simulink model "DAEMOT_Motor"  (R2025a)
settings: Solver=ode15s  StartTime=0.0  StopTime=10.0  RelTol=1e-3
undefined symbols (not defined in the file or in its folder): rev_comms_sink
settings Model: Creator=jmp8430  LastModifiedBy=jmp8430

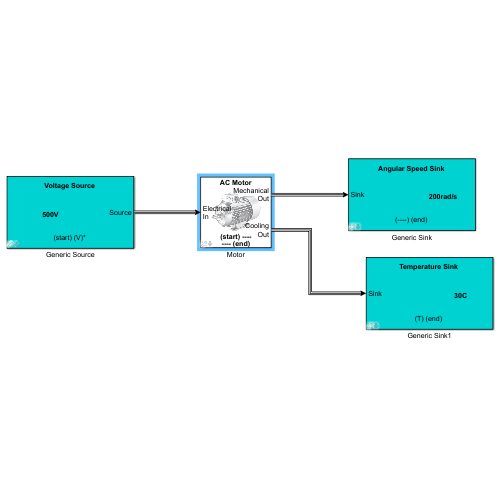
[thumbnail: Simulink's stored preview of the top-level diagram]
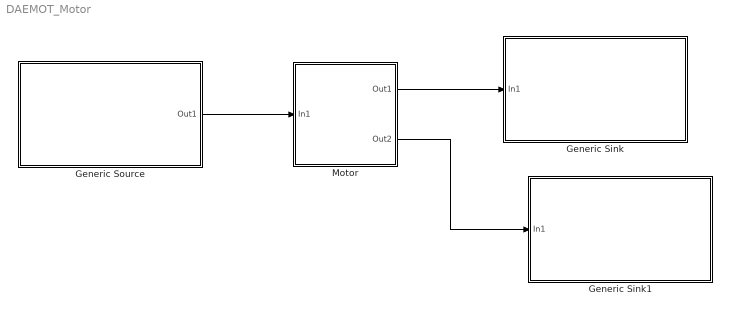
== system DAEMOT_Motor ==
  Generic Sink : Subsystem  AncestorBlock=DAEMOT_Lib/Support Functions/Generic Sink  mask(Effort Sink (Torque)){Stype=Angular Speed Sink, const=on, value=200}
      mask prompts: Stype "Sink Type"; const "Constant Value?"; value "Speed [rad/s]"
      mask help: Used to create a effot sink.
      mask init:
      | h      = get_param(gcb,'handle');   % Get block handle
      | blk    = gcb;
      | hblock = get(h);     % Parse out handles structure
      | 
      | if const == 1;
      |     try delete_block([blk,'/In2'])
      |         delete_unconnected_lines(blk);
      |         add_block('simulink/Sources/Constant',   [blk,'/val'], 'Position', [200,218,230,232]);
      |         add_line(blk,'val/1','Sink1/1','AutoRouting','on');
      |         set_param([blk,'/val'],'Value','value');
      |     end
      |      
      | %     delete_unconnected_lines(blk)
      | else
      |     try delete_block([blk,'/val'])
      |         delete_unconnected_lines(blk);
      |         add_block('simulink/Ports & Subsystems/In1',   [blk,'/In2'], 'Position', [200,218,230,232]);
      |         add_line(blk,'In2/1','Sink1/1','AutoRouting','on');
      |     end
      | end
      | 
      | clear h blk hblock
      settings: CopyFcn=|
      | h      = get_param(gcb,'handle');   % Get block handle
      | blk    = gcb;
      | 
      | set_param(blk, 'LinkStatus', 'inactive')
      | clear h
      | clear blk
      mask TypeOptions Stype: Voltage Sink | Current Sink | Angular Speed Sink | Torque Sink | Temperature Sink | Heat Flow Sink | Pressure Sink | Mass Flow Sink
      mask Callback Stype:
      | mp     = get_param(gcb,'MaskPrompts');
      | h      = get_param(gcb,'handle');   % Get block handle
      | blk    = gcb;
      | hblock = get(h);     % Parse out handles structure
      | 
      | switch get_param(gcb,'Stype')
      |     case 'Voltage Sink'
      |         mp{3} = 'Voltage [V]';
      |     case 'Current Sink'
      |         mp{3} = 'Current [A]';
      |     case 'Angular Speed Sink'
      |         mp{3} = 'Speed [rad/s]';
      |     case 'Torque Sink'
      |         mp{3} = 'Torque [Nm]';
      |     case 'Temperature Sink'
      |         mp{3} = 'Temperature [C]';
      |     case 'Heat Flow Sink'
      |         mp{3} = 'Heat Flow [kW]';
      |     case 'Pressure Sink'
      |         mp{3} = 'Pressure [kPa]';
      |     case 'Mass Flow Sink'
      |         mp{3} = 'Mass Flow [kg/s]';
      | end
      | set_param(gcb,'MaskPrompts',mp);
      | 
      | clear mp h blk hblock
      mask Callback const:
      | en = get_param(gcb,'MaskVisibilities');
      | h      = get_param(gcb,'handle');   % Get block handle
      | blk    = gcb;
      | hblock = get(h);     % Parse out handles structure
      | 
      | switch get_param(gcb,'const')
      |     case 'on'
      |         en{3} = 'on';
      | %         delete_block([blk,'/In1'])
      | 
      |     case 'off'
      |         en{3} = 'off';
      | %         add_block('simulink/Ports & Subsystems/In1',   [blk,'/In1'],'Position',[130    -7   160     7]);         % adding inport
      | 
      | end
      | set_param(gcb,'MaskVisibilities',en);
      | 
      | % hblock.MaskPrompts{3} = 'hello';
      | clear en h blk hblock
      mask Display:
      | text(0.5,0.90,['{\bf',get_param(gcb,'Stype'),'}'],'TexMode','on','horizontalAlignment', 'center')
      | % text(0.5,0.1,['{(T)(end)}'],'TexMode','on','horizontalAlignment', 'center')
      | 
      | type = get_param(gcb,'Stype');
      | switch type
      |         case 'Voltage Sink'
      |             nm = 'Voltage [V]';
      |             id = '(V)';
      |             un = 'V';
      |         case 'Current Sink'
      |             nm = 'Current [A]';
      |             id = '(----)';
      |             un = 'A';
      |         case 'Angular Speed Sink'
      |             nm = 'Speed [rad/s]';
      |             id = '(----)';
      |             un = 'rad/s';
      |         case 'Torque Sink'
      |             nm = 'Torque [Nm]';
      |             id = '(\tau)';
      |             un = 'Nm';
      |         case 'Temperature Sink'
      |             nm = 'Temperature [C]';
      |             id = '(T)';
      |             un = 'C';
      |         case 'Heat Flow Sink'
      |             nm = 'Heat Flow [kW]';
      |             id = '(----)';
      |             un = 'kW';
      |         case 'Pressure Sink'
      |             nm = 'Pressure [kPa]';
      |             id = '(P)';
      |             un = 'kPa';
      |         case 'Mass Flow Sink'
      |             nm = 'Mass Flow [kg/s]';
      |             id = '(----)';
      |             un = 'kg/s';
      | end
      | 
      | if strcmp(get_param(gcb,'const'),'on')
      |     text(0.75,0.500,['{\bf',get_param(gcb,'Value'),un,'}'],'TexMode','on','horizontalAlignment', 'center')
      | else
      |     port_label('input',2,sprintf(['Sink ',nm]));
      | end
      | 
      | 
      | port_label('input',1,'Sink');
      | text(0.5,0.175,['{',id,' (end)}'],'TexMode','on','horizontalAlignment', 'center');
  Generic Sink1 : Subsystem  AncestorBlock=DAEMOT_Lib/Support Functions/Generic Sink  mask(Effort Sink (Torque)){Stype=Temperature Sink, const=on, value=30}
      mask prompts: Stype "Sink Type"; const "Constant Value?"; value "Temperature [C]"
      mask help: Used to create a effot sink.
      mask init: same as DAEMOT_Motor/Generic Sink
      settings: CopyFcn=|
      | h      = get_param(gcb,'handle');   % Get block handle
      | blk    = gcb;
      | 
      | set_param(blk, 'LinkStatus', 'inactive')
      | clear h
      | clear blk
      mask TypeOptions Stype: Voltage Sink | Current Sink | Angular Speed Sink | Torque Sink | Temperature Sink | Heat Flow Sink | Pressure Sink | Mass Flow Sink
      mask Callback Stype:
      | mp     = get_param(gcb,'MaskPrompts');
      | h      = get_param(gcb,'handle');   % Get block handle
      | blk    = gcb;
      | hblock = get(h);     % Parse out handles structure
      | 
      | switch get_param(gcb,'Stype')
      |     case 'Voltage Sink'
      |         mp{3} = 'Voltage [V]';
      |     case 'Current Sink'
      |         mp{3} = 'Current [A]';
      |     case 'Angular Speed Sink'
      |         mp{3} = 'Speed [rad/s]';
      |     case 'Torque Sink'
      |         mp{3} = 'Torque [Nm]';
      |     case 'Temperature Sink'
      |         mp{3} = 'Temperature [C]';
      |     case 'Heat Flow Sink'
      |         mp{3} = 'Heat Flow [kW]';
      |     case 'Pressure Sink'
      |         mp{3} = 'Pressure [kPa]';
      |     case 'Mass Flow Sink'
      |         mp{3} = 'Mass Flow [kg/s]';
      | end
      | set_param(gcb,'MaskPrompts',mp);
      | 
      | clear mp h blk hblock
      mask Callback const:
      | en = get_param(gcb,'MaskVisibilities');
      | h      = get_param(gcb,'handle');   % Get block handle
      | blk    = gcb;
      | hblock = get(h);     % Parse out handles structure
      | 
      | switch get_param(gcb,'const')
      |     case 'on'
      |         en{3} = 'on';
      | %         delete_block([blk,'/In1'])
      | 
      |     case 'off'
      |         en{3} = 'off';
      | %         add_block('simulink/Ports & Subsystems/In1',   [blk,'/In1'],'Position',[130    -7   160     7]);         % adding inport
      | 
      | end
      | set_param(gcb,'MaskVisibilities',en);
      | 
      | % hblock.MaskPrompts{3} = 'hello';
      | clear en h blk hblock
      mask Display:
      | text(0.5,0.90,['{\bf',get_param(gcb,'Stype'),'}'],'TexMode','on','horizontalAlignment', 'center')
      | % text(0.5,0.1,['{(T)(end)}'],'TexMode','on','horizontalAlignment', 'center')
      | 
      | type = get_param(gcb,'Stype');
      | switch type
      |         case 'Voltage Sink'
      |             nm = 'Voltage [V]';
      |             id = '(V)';
      |             un = 'V';
      |         case 'Current Sink'
      |             nm = 'Current [A]';
      |             id = '(----)';
      |             un = 'A';
      |         case 'Angular Speed Sink'
      |             nm = 'Speed [rad/s]';
      |             id = '(----)';
      |             un = 'rad/s';
      |         case 'Torque Sink'
      |             nm = 'Torque [Nm]';
      |             id = '(\tau)';
      |             un = 'Nm';
      |         case 'Temperature Sink'
      |             nm = 'Temperature [C]';
      |             id = '(T)';
      |             un = 'C';
      |         case 'Heat Flow Sink'
      |             nm = 'Heat Flow [kW]';
      |             id = '(----)';
      |             un = 'kW';
      |         case 'Pressure Sink'
      |             nm = 'Pressure [kPa]';
      |             id = '(P)';
      |             un = 'kPa';
      |         case 'Mass Flow Sink'
      |             nm = 'Mass Flow [kg/s]';
      |             id = '(----)';
      |             un = 'kg/s';
      | end
      | 
      | if strcmp(get_param(gcb,'const'),'on')
      |     text(0.75,0.500,['{\bf',get_param(gcb,'Value'),un,'}'],'TexMode','on','horizontalAlignment', 'center')
      | else
      |     port_label('input',2,sprintf(['Sink ',nm]));
      | end
      | 
      | 
      | port_label('input',1,'Sink');
      | text(0.5,0.175,['{',id,' (end)}'],'TexMode','on','horizontalAlignment', 'center');
  Generic Source : Subsystem  AncestorBlock=DAEMOT_Lib/Support Functions/Generic Source  mask(Effort Source (Voltage)){Stype=Voltage Source, const=on, value=500}
      mask prompts: Stype "Source Type"; const "Constant Value?"; value "Voltage [V]"
      mask help: Used to create an effort source.
      mask init:
      | h      = get_param(gcb,'handle');   % Get block handle
      | blk    = gcb;
      | hblock = get(h);     % Parse out handles structure
      | type = get_param(gcb,'Stype');
      |         
      | switch type
      |     case 'Voltage Source'
      |         up = 'current';
      |         dw = 'voltage';
      |     case 'Current Source'
      |         dw = 'current';
      |         up = 'voltage';
      |     case 'Angular Speed Source'
      |         up = 'torque';
      |         dw = 'aspeed';
      |     case 'Torque Source'
      |         dw = 'torque';
      |         up = 'aspeed';
      |     case 'Temperature Source'
      |         up = 'Q_kW';
      |         dw = 'Temp';
      |     case 'Heat Flow Source'
      |         dw = 'Q_kW';
      |         up = 'Temp';
      |     case 'Pressure Source'
      |         up = 'mdot_kgps';
      |         mid= 'T_C';
      |         dw = 'P_kPa';
      |     case 'Mass Flow Source'
      |         up = 'P_kpa';
      |         mid= 'T_C';
      |         dw = 'mdot_kgps';
      |         %up = 'mdot_kgps';
      |         %mid= 'T_C';
      |         %dw = 'P_kPa';
      | end
      | 
      | if (((type(1) == 'P') || (type(1) == 'M')) && (const == 1)) %if constant input (user defined in mask) and need temperature input
      |     
      |     try add_block('simulink/Ports & Subsystems/In1', [blk,'/In2'], 'Position', [200,230,230,245]) %make temperature input
      |         set_param([blk, '/b1'],'Inputs','3');
      |         add_line(blk,'In2/1','b1/3','AutoRouting','on');
      |             
      |         p = get_param([blk,'/In2'],'PortHandles');
      |         l = get_param(p.Outport,'Line');
      |         set_param(l,'Name',mid);
      |     end 
      |     
      |     try delete_block([blk,'/In1'])
      |         delete_unconnected_lines(blk);
      |         
      |         fprintf ("option 1\n");        
      |         
      |         add_block('simulink/Sources/Constant',   [blk,'/val'], 'Position', [200,148,230,162]);
      |         add_line(blk,'val/1','b1/2','AutoRouting','on');
      |         set_param([blk,'/val'],'Value','value');
      |         
      |         p = get_param([blk,'/Constant'],'PortHandles');
      |         l = get_param(p.Outport,'Line');
      |         set_param(l,'Name',up);
      | 
      |         p = get_param([blk,'/val'],'PortHandles');
      |         l = get_param(p.Outport,'Line');
      |         set_param(l,'Name',dw);
      |         
      |     end
      |     p = get_param([blk,'/Constant'],'PortHandles');
      |     l = get_param(p.Outport,'Line');
      | 
      |     if (strcmp(get_param(l,'name'),up)) %If it didn't work and l's name doesn't match what it should, set them again.
      |     else
      |         set_param(l,'Name',up);
      |         
      |         fprintf ("failed strcmp \n");
      |                 
      |         p = get_param([blk,'/val'],'PortHandles');
      |         l = get_param(p.Outport,'Line');
      |         set_param(l,'Name',dw);
      |             
      |         p = get_param([blk,'/In2'],'PortHandles');
      |         l = get_param(p.Outport,'Line');
      |         set_param(l,'Name',mid);
      |     end
      |     
      | elseif ((type(1) == 'P') || (type(1) == 'M')) %if need input port (not user defined in mask) and also need temperature input
      |     
      |     try add_block('simulink/Ports & Subsystems/In1', [blk,'/In2'], 'Position', [200,230,230,245]) %make temperature input
      |         set_param([blk, '/b1'],'Inputs','3');
      |         add_line(blk,'In2/1','b1/3','AutoRouting','on');
      | 
      |         p = get_param([blk,'/In2'],'PortHandles');
      |         l = get_param(p.Outport,'Line');
      |         set_param(l,'Name',mid);
      |     end
      |     
      |     try delete_block([blk,'/val'])
      |         delete_unconnected_lines(blk);
      |         
      |         fprintf ("option 2\n");      
      |         
      |         add_block('simulink/Ports & Subsystems/In1', [blk,'/In1'], 'Position', [200,148,230,162]);
      |         add_line(blk,'In1/1','b1/2','AutoRouting','on');
      |         
      |         p = get_param([blk,'/Constant'],'PortHandles');
      |         l = get_param(p.Outport,'Line');
      |         set_param(l,'Name',up);
      | 
      |         p = get_param([blk,'/In1'],'PortHandles');
      |         l = get_param(p.Outport,'Line');
      |         set_param(l,'Name',dw);
      |         
      |     end
      |     
      |     p = get_param([blk,'/Constant'],'PortHandles');
      |     l = get_param(p.Outport,'Line');
      |     if (strcmp(get_param(l,'name'),up)) %If it didn't work and l's name doesn't match what it should, set them again.
      |     else
      |         set_param(l,'Name',up);
      |         
      |         fprintf ("failed strcmp \n");
      |         
      |         p = get_param([blk,'/In1'],'PortHandles');
      |         l = get_param(p.Outport,'Line');
      |         set_param(l,'Name',dw);
      | 
      |         p = get_param([blk,'/In2'],'PortHandles');
      |         l = get_param(p.Outport,'Line');
      |         set_param(l,'Name',mid);
      |     end
      |     
      | elseif (const == 1) %if constant, user-defined input, but does not need a temperature input port
      |     try delete_block([blk,'/In2']) %delete temperature input
      |         delete_unconnected_lines(blk);
      |         
      |         set_param([blk, '/b1'],'Inputs','2');
      |         fprintf ("delete in2 \n");
      |     end
      |     
      |     try delete_block([blk,'/In1'])
      |         delete_unconnected_lines(blk);
      |         
      |         fprintf ("option 3\n");
      |         
      |         add_block('simulink/Sources/Constant',   [blk,'/val'], 'Position', [200,198,230,212]);
      |         add_line(blk,'val/1','b1/2','AutoRouting','on');
      |         set_param([blk,'/val'],'Value','value');
      |         
      |         p = get_param([blk,'/Constant'],'PortHandles');
      |         l = get_param(p.Outport,'Line');
      |         set_param(l,'Name',up);
      |         
      |         p = get_param([blk,'/val'],'PortHandles');
      |         l = get_param(p.Outport,'Line');
      |         set_param(l,'Name',dw);
      |     end
      |     
      |     p = get_param([blk,'/Constant'],'PortHandles');
      |     l = get_param(p.Outport,'Line');
      |     if (strcmp(get_param(l,'name'),up))
      |     else
      |         set_param(l,'Name',up);
      |         
      |         fprintf ("failed strcmp \n");
      |                 
      |         p = get_param([blk,'/val'],'PortHandles');
      |         l = get_param(p.Outport,'Line');
      |         set_param(l,'Name',dw);
      |     end
      |     
      | else %if need an input port for the input, but not for temperature
      |     try delete_block([blk,'/In2']) %delete temperature input
      |         delete_unconnected_lines(blk);
      |         
      |         set_param([blk, '/b1'],'Inputs','2');
      |         fprintf ("deleted in2 \n");
      |     end    
      |         
      |     try delete_block([blk,'/val'])
      |         delete_unconnected_lines(blk);
      |         
      |         fprintf ("option 4\n");
      |         
      |         add_block('simulink/Ports & Subsystems/In1',   [blk,'/In1'], 'Position', [200,198,230,212]);
      |         add_line(blk,'In1/1','b1/2','AutoRouting','on');
      |         
      |         p = get_param([blk,'/Constant'],'PortHandles');
      |         l = get_param(p.Outport,'Line');
      |         set_param(l,'Name',up);
      | 
      |         p = get_param([blk,'/In1'],'PortHandles');
      |         l = get_param(p.Outport,'Line');
      |         set_param(l,'Name',dw);
      |     end
      |     
      |     p = get_param([blk,'/Constant'],'PortHandles');
      |     l = get_param(p.Outport,'Line');
      |     if (strcmp(get_param(l,'name'),up))
      |     else
      |         set_param(l,'Name',up);
      |         fprintf ("failed strcmp \n");
      |         p = get_param([blk,'/In1'],'PortHandles');
      |         l = get_param(p.Outport,'Line');
      |         set_param(l,'Name',dw);
      |     end
      |     
      | end
      | 
      | 
      | %if const == 1;
      | %    try delete_block([blk,'/In1'])
      | %        delete_unconnected_lines(blk);
      | %        add_block('simulink/Sources/Constant',   [blk,'/val'], 'Position', [200,198,230,212]);
      | %        add_line(blk,'val/1','b1/2','AutoRouting','on');
      | %        set_param([blk,'/val'],'Value','value');
      | 
      | %        p = get_param([blk,'/Constant'],'PortHandles');
      | %        l = get_param(p.Outport,'Line');
      | %        set_param(l,'Name',up);
      |         
      | %        p = get_param([blk,'/val'],'PortHandles');
      | %        l = get_param(p.Outport,'Line');
      | %        set_param(l,'Name',dw);
      | %    end
      | %    p = get_param([blk,'/Constant'],'PortHandles');
      | %    l = get_param(p.Outport,'Line');
      | %    if strcmp(get_param(l,'name'),up)
      | %    else
      | %       set_param(l,'Name',up);
      |         
      | %        p = get_param([blk,'/val'],'PortHandles');
      | %        l = get_param(p.Outport,'Line');
      | %        set_param(l,'Name',dw);
      | %    end
      |      
      | %%     delete_unconnected_lines(blk)
      | %else
      | %    try delete_block([blk,'/val'])
      | %        delete_unconnected_lines(blk);
      | %        add_block('simulink/Ports & Subsystems/In1',   [blk,'/In1'], 'Position', [200,198,230,212]);
      | %        add_line(blk,'In1/1','b1/2','AutoRouting','on');
      |         
      | %        p = get_param([blk,'/Constant'],'PortHandles');
      | %        l = get_param(p.Outport,'Line');
      | %        set_param(l,'Name',up);
      | 
      | %        p = get_param([blk,'/In1'],'PortHandles');
      | %        l = get_param(p.Outport,'Line');
      | %        set_param(l,'Name',dw);
      | %    end
      | %    p = get_param([blk,'/Constant'],'PortHandles');
      | %    l = get_param(p.Outport,'Line');
      | %    if strcmp(get_param(l,'name'),up)
      | %    else
      | %        set_param(l,'Name',up);
      |         
      | %        p = get_param([blk,'/In1'],'PortHandles');
      | %        l = get_param(p.Outport,'Line');
      | %        set_param(l,'Name',dw);
      | %    end
      | %end
      | 
      | clear h blk hblock type
      settings: CopyFcn=|
      | h      = get_param(gcb,'handle');   % Get block handle
      | blk    = gcb;
      | 
      | set_param(blk, 'LinkStatus', 'inactive')
      | clear h
      | clear blk
      mask TypeOptions Stype: Voltage Source | Current Source | Angular Speed Source | Torque Source | Temperature Source | Heat Flow Source | Pressure Source | Mass Flow Source
      mask Callback Stype:
      | mp     = get_param(gcb,'MaskPrompts');
      | h      = get_param(gcb,'handle');   % Get block handle
      | blk    = gcb;
      | hblock = get(h);     % Parse out handles structure
      | 
      | switch get_param(gcb,'Stype')
      |     case 'Voltage Source'
      |         mp{3} = 'Voltage [V]';
      |     case 'Current Source'
      |         mp{3} = 'Current [A]';
      |     case 'Angular Speed Source'
      |         mp{3} = 'Speed [rad/s]';
      |     case 'Torque Source'
      |         mp{3} = 'Torque [Nm]';
      |     case 'Temperature Source'
      |         mp{3} = 'Temperature [C]';
      |     case 'Heat Flow Source'
      |         mp{3} = 'Heat Flow [kW]';
      |     case 'Pressure Source'
      |         mp{3} = 'Pressure [kPa]';
      |     case 'Mass Flow Source'
      |         mp{3} = 'Mass Flow [kg/s]';
      | end
      | set_param(gcb,'MaskPrompts',mp);
      | 
      | clear mp h blk hblock
      mask Callback const:
      | en = get_param(gcb,'MaskVisibilities');
      | h      = get_param(gcb,'handle');   % Get block handle
      | blk    = gcb;
      | hblock = get(h);     % Parse out handles structure
      | 
      | switch get_param(gcb,'const')
      |     case 'on'
      |         en{3} = 'on';
      | %         delete_block([blk,'/In1'])
      | 
      |     case 'off'
      |         en{3} = 'off';
      | %         add_block('simulink/Ports & Subsystems/In1',   [blk,'/In1'],'Position',[130    -7   160     7]);         % adding inport
      | 
      | end
      | set_param(gcb,'MaskVisibilities',en);
      | 
      | % hblock.MaskPrompts{3} = 'hello';
      | clear en h blk hblock
      mask Display:
      | text(0.5,0.900,['{\bf',get_param(gcb,'Stype'),'}'],'TexMode','on','horizontalAlignment', 'center')
      | 
      | type = get_param(gcb,'Stype');
      | switch type
      |     case 'Voltage Source'
      |         nm = 'Voltage [V]';
      |         id = '(V)*';
      |         un = 'V';
      |     case 'Current Source'
      |         nm = 'Current [A]';
      |         id = '(----)';
      |         un = 'A';
      |     case 'Angular Speed Source'
      |         nm = 'Speed [rad/s]';
      |         id = '(----)';
      |         un = 'rad/s';
      |     case 'Torque Source'
      |         nm = 'Torque [Nm]';
      |         id = '(\tau)*';
      |         un = 'Nm';
      |     case 'Temperature Source'
      |         nm = 'Temperature [C]';
      |         id = '(T)';
      |         un = 'C';
      |     case 'Heat Flow Source'
      |         nm = 'Heat Flow [kW]';
      |         id = '(----)';
      |         un = 'kW';
      |     case 'Pressure Source'
      |         nm = 'Pressure [kPa]';
      |         id = '(P)';
      |         un = 'kPa';
      |     case 'Mass Flow Source'
      |         nm = 'Mass Flow [kg/s]';
      |         id = '(----)';
      |         un = 'kg/s';
      | end
      | 
      | if strcmp(get_param(gcb,'const'),'on')
      |     text(0.35,0.500,['{\bf',get_param(gcb,'Value'),un,'}'],'TexMode','on','horizontalAlignment', 'center')
      | else
      |     port_label('input',1,sprintf(['Source \n',nm]))
      | end
      | port_label('output',1,'Source')
      | text(0.5,0.175,['{(start) ',id,'}'],'TexMode','on','horizontalAlignment', 'center')
      | 
      | switch type
      |     case 'Pressure Source'
      |         if strcmp(get_param(gcb,'const'),'off')
      |             port_label('input',2,sprintf(['Source\nTemp. [C]']))
      |         else
      |             port_label('input',1,sprintf(['Source\nTemp. [C]']))
      | 
      |         end
      |     case 'Mass Flow Source'
      |         if strcmp(get_param(gcb,'const'),'off')
      |             port_label('input',2,sprintf(['Source\nTemp. [C]']))
      |         else
      |             port_label('input',1,sprintf(['Source\nTemp. [C]']))
      | 
      |         end
      | end
  Motor : Subsystem  AncestorBlock=DAEMOT_Lib/Electrical/Motor  mask{m_type=AC, R=0.013461960749493, Kv=0.009688163543703, c=0.000234355495215172, b=1.89435163576232e-05, L=1.252192537082724e-05, J=1.09*10^-4, I_initial=1, w_initial=1, Cp=60, T_initial=25}
      mask prompts: m_type "Motor Type"; R "Armature Resistance [Ohm]"; Kv "Motor Constant [Nm/A] or [V-s/rad]"; c "Static Friction Coefficient [Nm]"; b "Viscous Friction Coefficient [N*m*s/rad]"; L "Armature Inductance [H]"; J "Shaft Inertia [kg*m^2]"; I_initial "Initial Total Current [A]"; w_initial "Initial Speed [rad/s]"; Cp "Motor Heat Capacity [J/K]"; T_initial "Initial Temperature [C]"
      settings: LibrarySourceBlock=DAEMOT_Lib_Copy/Dyn Electrical Comp/Motor
      settings: CopyFcn=|
      | h      = get_param(gcb,'handle');   % Get block handle
      | blk    = gcb;
      | 
      | set_param(blk, 'LinkStatus', 'inactive')
      | clear h
      | clear blk
      mask TypeOptions m_type: DC | AC
      mask DialogControl ParameterTabVar0 Prompt: Motor Parameters
      mask DialogControl ParameterTabVar01 Prompt: Cooling
      mask DialogControl ParameterTabVar012 Prompt: System
      mask Display:
      | image(imread('motor.bmp'));
      | T = get_param(gcb,'m_type');
      | if strcmp(T,'DC')
      |     text(0.5,0.95,['{\bf DC Motor}'],'TexMode','on','horizontalAlignment', 'center')
      | else
      |     text(0.5,0.95,['{\bf AC Motor}'],'TexMode','on','horizontalAlignment', 'center')
      | end
      | text(0.5,0.075,['{\bf ---- (end)}'],'TexMode','on','horizontalAlignment', 'center')
      | text(0.5,0.175,['{\bf (start) ----}'],'TexMode','on','horizontalAlignment', 'center')
      | 
      | port_label('input',1,sprintf('Electrical \nIn'))
      | port_label('output',1,sprintf('Mechanical \nOut'))
      | port_label('output',2,sprintf('Cooling \nOut'))
  wires:
  Motor/1(Out1) -> Generic Sink/1(In1)
  Motor/2(Out2) -> Generic Sink1/1(In1)
  Generic Source/1(Out1) -> Motor/1(In1)

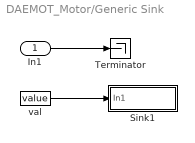
== system DAEMOT_Motor/Generic Sink ==
  In1 : Inport
  Sink1 : Subsystem  LoadFcn=rev_comms_sink();  InitFcn=rev_comms_sink();  mask(Sink){}
      mask help: Used for sending data to the upstream component.
      settings: CopyFcn=rev_comms_sink();  NameChangeFcn=rev_comms_sink();
      mask Display: text(0.25,0.5,'Sink')
  Terminator : Terminator
  val : Constant  Value=value
  wires:
  val/1 -> Sink1/1(In1)
  In1/1 -> Terminator/1

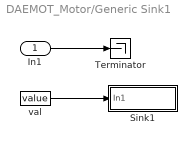
== system DAEMOT_Motor/Generic Sink1 ==
  In1 : Inport
  Sink1 : Subsystem  LoadFcn=rev_comms_sink();  InitFcn=rev_comms_sink();  mask(Sink){}
      mask help: Used for sending data to the upstream component.
      settings: CopyFcn=rev_comms_sink();  NameChangeFcn=rev_comms_sink();
      mask Display: text(0.25,0.5,'Sink')
  Terminator : Terminator
  val : Constant  Value=value
  wires:
  val/1 -> Sink1/1(In1)
  In1/1 -> Terminator/1

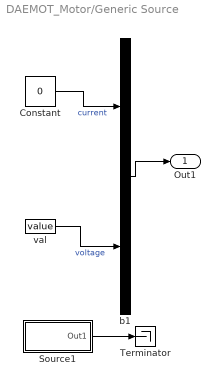
== system DAEMOT_Motor/Generic Source ==
  Constant : Constant  Value=0
  Source1 : Subsystem  mask(Source){}
      mask help: Used for receiving data from the downstream component.
      mask init:
      | n_src = gcb;
      | n_src = str2num(n_src(end));
      | try
      |     rev_comms_source(n_src);
      | catch
      | 
      | end
      mask Display: text(0.25,0.5,'Source')
  Terminator : Terminator
  b1 : BusCreator  Inputs=2
  val : Constant  Value=value
  Out1 : Outport  VectorParamsAs1DForOutWhenUnconnected=off
  wires:
  val/1 -> b1/2  "voltage"
  b1/1 -> Out1/1
  Source1/1(Out1) -> Terminator/1
  Constant/1 -> b1/1  "current"

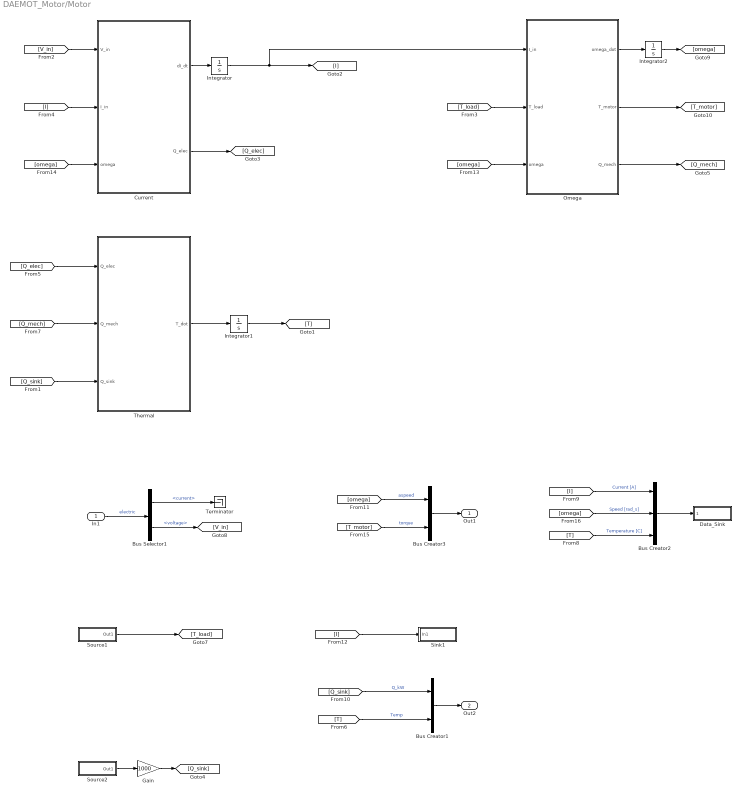
== system DAEMOT_Motor/Motor ==
  In1 : Inport
  Bus Creator1 : BusCreator  Inputs=2
  Bus Creator2 : BusCreator  Inputs=3
  Bus Creator3 : BusCreator  Inputs=2
  Bus Selector1 : BusSelector  OutputSignals=current,voltage
  Current : MATLAB Function  TreatAsAtomicUnit=on
  Data_Sink : Subsystem  LoadFcn=|  InitFcn=|  mask(Data Sink){}
      LoadFcn=|
      | h      = get_param(gcb,'handle');   % Get block handle                           
      | hblock = get(h);     % Parse out handles structure
      | 
      | str = [hblock.Path(numel(bdroot)+2:end), hblock.Name];
      | str(~ismember(str,['A':'Z' 'a':'z' '0':'9' '_'])) = '';                     
      | set_param([gcb, '/global_data_goto'],'GotoTag',['gdata_',str]);
      |                                
      |                                                                                  
      | clear h hblock str
      InitFcn=|
      | h      = get_param(gcb,'handle');   % Get block handle                           
      | hblock = get(h);     % Parse out handles structure
      | 
      | str = [hblock.Path(numel(bdroot)+2:end), hblock.Name];
      | str(~ismember(str,['A':'Z' 'a':'z' '0':'9' '_'])) = '';                     
      | set_param([gcb, '/global_data_goto'],'GotoTag',['gdata_',str]);
      |                                
      |                                                                                  
      | clear h hblock str
      mask help:
      | Input to this block should be a bus signal with named signals.
      |
      | Bus signals sent to this block will be read by the Data Manager.
      | The Data Manager will handle the global routing of signals.
      |
      | This block should be placed under the mask of components.
      settings: CopyFcn=|
      | h      = get_param(gcb,'handle');   % Get block handle
      | hblock = get(h);     % Parse out handles structure
      | 
      | str = [hblock.Path(numel(bdroot)+2:end), hblock.Name];
      | str(~ismember(str,['A':'Z' 'a':'z' '0':'9' '_'])) = '';
      | set_param([gcb, '/global_data_goto'],'GotoTag',['gdata_',str]);
      | 
      | 
      | clear h hblock str
      settings: NameChangeFcn=|
      | h      = get_param(gcb,'handle');   % Get block handle
      | hblock = get(h);     % Parse out handles structure
      | 
      | str = [hblock.Path(numel(bdroot)+2:end), hblock.Name];
      | str(~ismember(str,['A':'Z' 'a':'z' '0':'9' '_'])) = '';
      | set_param([gcb, '/global_data_goto'],'GotoTag',['gdata_',str]);
      | 
      | 
      | clear h hblock str
      mask Display: text(0.25,0.5,'Data Sink')
  Gain : Gain  Gain=1000
  Integrator : Integrator  InitialCondition=I_initial
  Integrator1 : Integrator  InitialCondition=T_initial
  Integrator2 : Integrator  InitialCondition=w_initial
  Omega : MATLAB Function  TreatAsAtomicUnit=on
  Sink1 : Subsystem  LoadFcn=rev_comms_sink();  InitFcn=rev_comms_sink();  mask(Sink){}
      mask help: Used for sending data to the upstream component.
      settings: CopyFcn=rev_comms_sink();  NameChangeFcn=rev_comms_sink();
      mask Display: text(0.25,0.5,'Sink')
  Source1 : Subsystem  mask(Source){}
      mask help: Used for receiving data from the downstream component.
      mask init:
      | n_src = gcb;
      | n_src = str2num(n_src(end));
      | try
      |     rev_comms_source(n_src);
      | catch
      | 
      | end
      mask Display: text(0.25,0.5,'Source')
  Source2 : Subsystem  mask(Source){}
      mask help: Used for receiving data from the downstream component.
      mask init:
      | n_src = gcb;
      | n_src = str2num(n_src(end));
      | try
      |     rev_comms_source(n_src);
      | catch
      | 
      | end
      mask Display: text(0.25,0.5,'Source')
  Terminator : Terminator
  Thermal : MATLAB Function  TreatAsAtomicUnit=on
  Out1 : Outport
  Out2 : Outport  Port=2
  wires:
  Gain/1 -> [Q_sink]
  [Q_sink] -> Bus Creator1/1  "Q_kW"
  [T] -> Bus Creator1/2  "Temp"
  Bus Creator1/1 -> Out2/1
  [Q_mech] -> Thermal/2(Q_mech)
  Omega/3(Q_mech) -> [Q_mech]
  [omega] -> Omega/3(omega)
  Source1/1(Out1) -> [T_load]
  Source2/1(Out1) -> Gain/1
  [V_in] -> Current/1(V_in)
  Integrator/1 -> [I], Omega/1(I_in)
  [T] -> Bus Creator2/3  "Temperature [C]"
  [omega] -> Bus Creator2/2  "Speed [rad_s]"
  Bus Creator2/1 -> Data_Sink/1(" ")
  [omega] -> Current/3(omega)
  Bus Selector1/1 -> Terminator/1  "<current>"
  Bus Selector1/2 -> [V_in]  "<voltage>"
  [omega] -> Bus Creator3/1  "aspeed"
  [I] -> Sink1/1(In1)
  In1/1 -> Bus Selector1/1  "electric"
  Bus Creator3/1 -> Out1/1
  Current/1(dI_dt) -> Integrator/1
  [I] -> Current/2(I_in)
  Thermal/1(T_dot) -> Integrator1/1
  Integrator1/1 -> [T]
  Current/2(Q_elec) -> [Q_elec]
  [Q_elec] -> Thermal/1(Q_elec)
  [Q_sink] -> Thermal/3(Q_sink)
  Omega/1(omega_dot) -> Integrator2/1
  [T_load] -> Omega/2(T_load)
  Integrator2/1 -> [omega]
  Omega/2(T_motor) -> [T_motor]
  [T_motor] -> Bus Creator3/2  "torque"
  [I] -> Bus Creator2/1  "Current [A]"

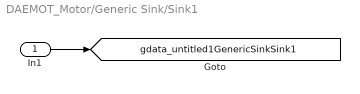
== system DAEMOT_Motor/Generic Sink/Sink1 ==
  In1 : Inport
  tag scope: gdata_untitled1GenericSinkSink1=global
  wires:
  In1/1 -> [gdata_untitled1GenericSinkSink1]

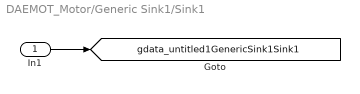
== system DAEMOT_Motor/Generic Sink1/Sink1 ==
  In1 : Inport
  tag scope: gdata_untitled1GenericSink1Sink1=global
  wires:
  In1/1 -> [gdata_untitled1GenericSink1Sink1]

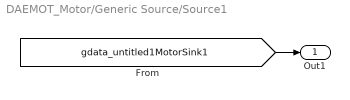
== system DAEMOT_Motor/Generic Source/Source1 ==
  Out1 : Outport  VectorParamsAs1DForOutWhenUnconnected=off
  wires:
  [gdata_untitled1MotorSink1] -> Out1/1

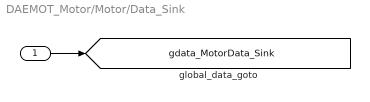
== system DAEMOT_Motor/Motor/Data_Sink ==
  " " : Inport
  tag scope: gdata_MotorData_Sink=global
  wires:
  " "/1 -> [gdata_MotorData_Sink]

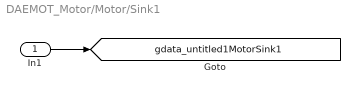
== system DAEMOT_Motor/Motor/Sink1 ==
  In1 : Inport
  tag scope: gdata_untitled1MotorSink1=global
  wires:
  In1/1 -> [gdata_untitled1MotorSink1]

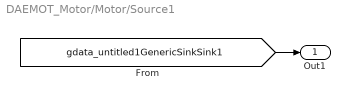
== system DAEMOT_Motor/Motor/Source1 ==
  Out1 : Outport
  wires:
  [gdata_untitled1GenericSinkSink1] -> Out1/1

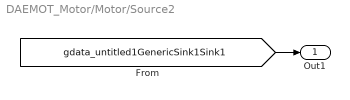
== system DAEMOT_Motor/Motor/Source2 ==
  Out1 : Outport
  wires:
  [gdata_untitled1GenericSink1Sink1] -> Out1/1

== matlab function DAEMOT_Motor/Motor/Current ==
  data: V_in input; I_in input; Kv parameter; R parameter; L parameter; omega input; dI_dt output; Q_elec output
function [dI_dt,Q_elec]= current(V_in,I_in,Kv, R, L,omega)


dI_dt = (1/L) * (V_in - R*I_in - Kv*omega);

Q_elec = R*I_in^2;

== matlab function DAEMOT_Motor/Motor/Omega ==
  data: I_in input; T_load input; omega_dot output; Kv parameter; omega input; T_motor output; J parameter; b parameter; c parameter; Q_mech output
function [omega_dot,T_motor,Q_mech]= omega(I_in,T_load,Kv,omega,J, b,c)

T_motor = Kv*I_in;

omega_dot = (1/(J))*(T_motor - T_load - b*omega - c*(2./(1+exp(-5*omega)) - 1));
Q_mech = b*omega^2 + c*omega*(2./(1+exp(-5*omega)) - 1);

== matlab function DAEMOT_Motor/Motor/Thermal ==
  data: Q_elec input; Q_mech input; T_dot output; Q_sink input; Cp parameter
function T_dot = Thermal(Q_elec,Q_mech, Q_sink, Cp)
%% Load Temperature
T_dot = (1/Cp) * (Q_elec + Q_mech - Q_sink);
